simulink model "HEVModel"  (R2021a)
settings: Solver=ode4  StartTime=0  StopTime=tEnd  FixedStep=dt  RelTol=1e-3
values from neighbouring files (symbols this model uses):
  accessoryLoad = 600    [main.m]
  Af = 1.00    (= 1)    [main.m]
  batteryCapacity = 50    [main.m]
  batteryResistance = 0.0461    [main.m]
  C = 400    [main.m]
  Cd = 0.576    [main.m]
  Crr = 0.01    [main.m]
  cycleNum = 2    [main.m]
  EffTableEff = [.75 .85 .89 .95 .96 .97 .98 .99 .99]    [main.m]
  EffTableSpeed = [0 5 10 15 25 35 45 55 65]    [main.m]
  etaGenGR = 0.93    [main.m]
  g = 9.81    [main.m]
  genMotorData = load(GENERATOR_MOTOR_DATA_NAME)    [main.m]
  GRd = 9.843    [main.m]
  GRgen = 1.4    [main.m]
  initialGasVolume = 5    [main.m]
  k_gal2kWh = 32.3    [main.m]
  k_hr2s = 3600    [main.m]
  k_J2gal = 1/3600000/32.3    (= 8.59993120055e-09)    [main.m]
  k_kW2W = 1000    [main.m]
  k_kWh2J = 3.6*10^6    (= 3600000)    [main.m]
  k_m2mi = 0.000621371    [main.m]
  k_m32gal = 264.172    [main.m]
  k_rpm2rps = 2*pi()/60    [main.m]
  k_rps2rpm = 60/(2*pi)    (= 9.54929658551)    [main.m]
  k_s2h = 1/3600    (= 0.000277777777778)    [main.m]
  k_W2kW = 1/1000    (= 0.001)    [main.m]
  kc = 0.513    [main.m]
  Kd = 0    [main.m]
  Ki = 0.1    [main.m]
  ki = 0.0773    [main.m]
  Kp = 200    [main.m]
  kw = 0.0000064    (= 6.4e-06)    [main.m]
  m = 1965    [main.m]
  motorMaxPower = 310000    [main.m]
  motorMaxSpeed = 18000    [main.m]
  motorMaxTorque = 600    [main.m]
  openCircuitVoltage = 420    [main.m]
  pBrakeMax = 4*TbrakeMax / (mu_k*pi()* cylinderBore^2 *meanPadRadius*numPads)    [main.m]
  r = 0.290    (= 0.29)    [main.m]
  rho = 1.20    (= 1.2)    [main.m]
  SOCi = 90    [main.m]
  theta = 0    [main.m]
  v0 = 0    [main.m]
  x0 = 0    [main.m]
libraries: autolibshared x6, fl_lib x5, nesl_utility x5, sdl_lib x1, autolibsharedmappedengines x1
(part 1 of 3)
settings Model: Creator=Chris  LastModifiedBy=jordan
settings SolverCC: AlgebraicLoopSolver=TrustRegion
settings DebuggingCC: SFMachineParentedDataDiag=warning

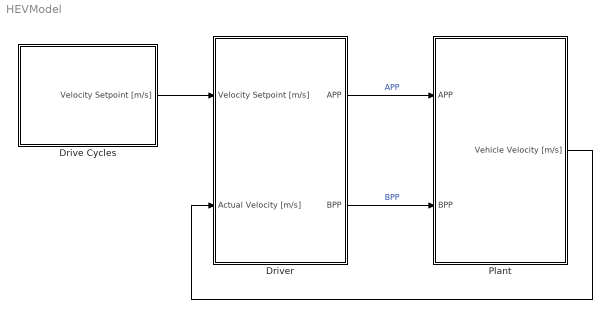
== system HEVModel ==
  Drive Cycles : Subsystem
  Driver : Subsystem
  Plant : Subsystem
  wires:
  Drive Cycles/1(Velocity Setpoint [m/s]) -> Driver/1(Velocity Setpoint [m/s])
  Driver/1(APP) -> Plant/1(APP)  "APP"
  Driver/2(BPP) -> Plant/2(BPP)  "BPP"
  Plant/1(Vehicle Velocity [m/s]) -> Driver/2(Actual Velocity [m/s])

== system HEVModel/Drive Cycles ==
  Constant : Constant  Value=cycleNum
  Drive Cycle Source1 : autolibshared/Drive Cycle Source  cycleVar=FTP75  wsVar=driveCycle  fileVar=cycleFTP75.mat  tfinal="2474  seconds"  cycleRepeat=off  outAccPort=off  outGearPort=off  gearList=No gear data  t_wot1=5  xdot_woto=0  xdot_wot1=30  t_wot2=20  xdot_wot2=0  t_wotend=30  srcUnit=m/s  outUnit=m/s  srcAccUnit=m/s/s  outAccUnit=m/s^2  dt=0  aMode=1  faultOption=off  velBnd=2  velBndUnit=mph  inUnit=m/s  timeBnd=1  failOption=off  stopSim=off  maxFaultCnt=10  maxFaultTime=2  maxTotFaultTime=15  traceOption=off  dtTrace=1  traceWindow=10  lastDCname=FTP75  lastOutUnit=mph  lastDT=0  lastTB=1  lastSB=2  forceCalcBound=off
      settings: SourceProductBaseCode=PW,DR,MT,UV,VE
  Drive Cycle Source2 : autolibshared/Drive Cycle Source  cycleVar=FTP75  wsVar=driveCycle  fileVar=cycleFTP75.mat  tfinal="2474  seconds"  cycleRepeat=off  outAccPort=off  outGearPort=off  gearList=No gear data  t_wot1=5  xdot_woto=0  xdot_wot1=30  t_wot2=20  xdot_wot2=0  t_wotend=30  srcUnit=m/s  outUnit=m/s  srcAccUnit=m/s/s  outAccUnit=m/s^2  dt=0  aMode=1  faultOption=off  velBnd=2  velBndUnit=mph  inUnit=m/s  timeBnd=1  failOption=off  stopSim=off  maxFaultCnt=10  maxFaultTime=2  maxTotFaultTime=15  traceOption=off  dtTrace=1  traceWindow=10  lastDCname=FTP75  lastOutUnit=mph  lastDT=0  lastTB=1  lastSB=2  forceCalcBound=off
      settings: SourceProductBaseCode=PW,DR,MT,UV,VE
  Drive Cycle Source3 : autolibshared/Drive Cycle Source  cycleVar=FTP75  wsVar=driveCycle  fileVar=cycleFTP75.mat  tfinal="2474  seconds, Cyclic"  cycleRepeat=on  outAccPort=off  outGearPort=off  gearList=No gear data  t_wot1=5  xdot_woto=0  xdot_wot1=30  t_wot2=20  xdot_wot2=0  t_wotend=30  srcUnit=m/s  outUnit=m/s  srcAccUnit=m/s/s  outAccUnit=m/s^2  dt=0  aMode=1  faultOption=off  velBnd=2  velBndUnit=mph  inUnit=m/s  timeBnd=1  failOption=off  stopSim=off  maxFaultCnt=10  maxFaultTime=2  maxTotFaultTime=15  traceOption=off  dtTrace=1  traceWindow=10  lastDCname=FTP75  lastOutUnit=mph  lastDT=0  lastTB=1  lastSB=2  forceCalcBound=off
      settings: SourceProductBaseCode=PW,DR,MT,UV,VE
  Drive Cycle Source4 : autolibshared/Drive Cycle Source  cycleVar=FTP75  wsVar=driveCycle  fileVar=cycleFTP75.mat  tfinal="2474  seconds, Cyclic"  cycleRepeat=on  outAccPort=off  outGearPort=off  gearList=No gear data  t_wot1=1  xdot_woto=0  xdot_wot1=30  t_wot2=tBrake  xdot_wot2=0  t_wotend=tWOTEnd  srcUnit=m/s  outUnit=m/s  srcAccUnit=m/s/s  outAccUnit=m/s^2  dt=0  aMode=1  faultOption=off  velBnd=2  velBndUnit=mph  inUnit=m/s  timeBnd=1  failOption=off  stopSim=off  maxFaultCnt=10  maxFaultTime=2  maxTotFaultTime=15  traceOption=off  dtTrace=1  traceWindow=10  lastDCname=FTP75  lastOutUnit=mph  lastDT=0  lastTB=1  lastSB=2  forceCalcBound=off
      settings: SourceProductBaseCode=PW,DR,MT,UV,VE
  Drive Cycle Source5 : autolibshared/Drive Cycle Source  cycleVar=FTP75  wsVar=driveCycle  fileVar=cycleFTP75.mat  tfinal="2474  seconds"  cycleRepeat=off  outAccPort=off  outGearPort=off  gearList=No gear data  t_wot1=5  xdot_woto=0  xdot_wot1=30  t_wot2=20  xdot_wot2=0  t_wotend=30  srcUnit=m/s  outUnit=m/s  srcAccUnit=m/s/s  outAccUnit=m/s^2  dt=0  aMode=1  faultOption=off  velBnd=2  velBndUnit=mph  inUnit=m/s  timeBnd=1  failOption=off  stopSim=off  maxFaultCnt=10  maxFaultTime=2  maxTotFaultTime=15  traceOption=off  dtTrace=1  traceWindow=10  lastDCname=FTP75  lastOutUnit=mph  lastDT=0  lastTB=1  lastSB=2  forceCalcBound=off
      settings: SourceProductBaseCode=PW,DR,MT,UV,VE
  Drive Cycle Source6 : autolibshared/Drive Cycle Source  cycleVar=Wide Open Throttle (WOT)  wsVar=driveCycle  fileVar=cycleFTP75.mat  tfinal="15  seconds, Cyclic"  cycleRepeat=on  outAccPort=off  outGearPort=off  gearList=No gear data  t_wot1=1  xdot_woto=0  xdot_wot1=vRef  t_wot2=tBrake2  xdot_wot2=-50  t_wotend=tEndWOT2  srcUnit=mph  outUnit=m/s  srcAccUnit=m/s/s  outAccUnit=m/s^2  dt=0  aMode=1  faultOption=off  velBnd=2  velBndUnit=mph  inUnit=m/s  timeBnd=1  failOption=off  stopSim=off  maxFaultCnt=10  maxFaultTime=2  maxTotFaultTime=15  traceOption=off  dtTrace=1  traceWindow=10  lastDCname=Custom Data Set  lastOutUnit=mph  lastDT=0  lastTB=1  lastSB=2  forceCalcBound=off
      settings: SourceProductBaseCode=PW,DR,MT,UV,VE
  Multiport Switch : MultiPortSwitch  Inputs=6
  Velocity Setpoint [m/s] : Outport
  wires:
  Drive Cycle Source6/1 -> Multiport Switch/7
  Drive Cycle Source5/1 -> Multiport Switch/6
  Drive Cycle Source4/1 -> Multiport Switch/4
  Drive Cycle Source1/1 -> Multiport Switch/5
  Drive Cycle Source2/1 -> Multiport Switch/2
  Constant/1 -> Multiport Switch/1
  Multiport Switch/1 -> Velocity Setpoint [m/s]/1  "Velocity Setpoint [m/s]"
  Drive Cycle Source3/1 -> Multiport Switch/3

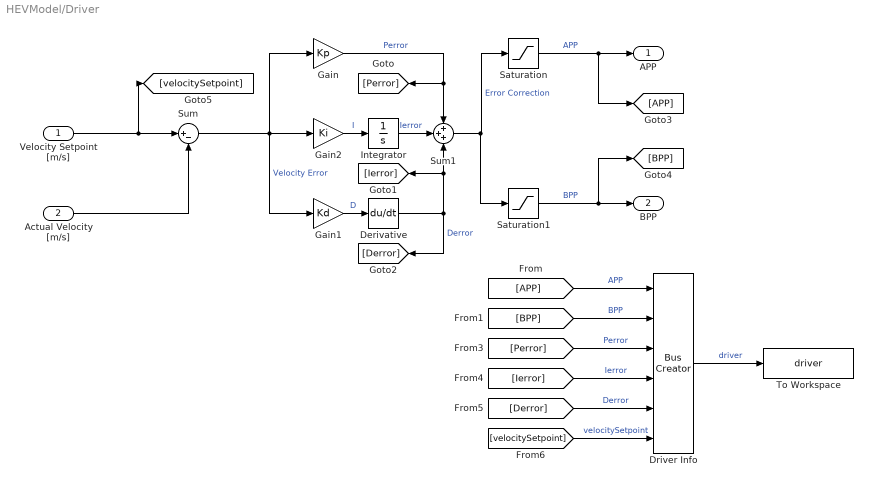
== system HEVModel/Driver ==
  Velocity Setpoint [m/s] : Inport
  Actual Velocity [m/s] : Inport  Port=2
  Derivative : Derivative
  Driver Info : BusCreator  Inputs=6
  Gain : Gain  Gain=Kp
  Gain1 : Gain  Gain=Kd
  Gain2 : Gain  Gain=Ki
  Integrator : Integrator
  Saturation : Saturate  UpperLimit=100  LowerLimit=0
  Saturation1 : Saturate  UpperLimit=0  LowerLimit=-100
  Sum : Sum  Inputs=|+-
  Sum1 : Sum  Inputs=+++
  To Workspace : ToWorkspace  VariableName=driver  SaveFormat=Timeseries  SampleTime=-1
  APP : Outport
  BPP : Outport  Port=2
  wires:
  Gain/1 -> [Perror], Sum1/1  "Perror"
  Integrator/1 -> Sum1/2  "Ierror"
  Derivative/1 -> [Derror], [Ierror], Sum1/3  "Derror"
  Sum1/1 -> Saturation1/1, Saturation/1  "Error Correction"
  Sum/1 -> Gain2/1, Gain1/1, Gain/1  "Velocity Error"
  Velocity Setpoint [m/s]/1 -> [velocitySetpoint], Sum/1
  Actual Velocity [m/s]/1 -> Sum/2
  Saturation1/1 -> [BPP], BPP/1  "BPP"
  Saturation/1 -> [APP], APP/1  "APP"
  Gain2/1 -> Integrator/1  "I"
  Gain1/1 -> Derivative/1  "D"
  Driver Info/1 -> To Workspace/1  "driver"
  [APP] -> Driver Info/1  "APP"
  [BPP] -> Driver Info/2  "BPP"
  [Perror] -> Driver Info/3  "Perror"
  [Ierror] -> Driver Info/4  "Ierror"
  [Derror] -> Driver Info/5  "Derror"
  [velocitySetpoint] -> Driver Info/6  "velocitySetpoint"

== system HEVModel/Plant ==
  APP : Inport
  BPP : Inport  Port=2
  Battery : Subsystem
  Brakes : Subsystem
  Driveline : Subsystem
  Fuel Tank Volume [gal] : Display
  Genset : Subsystem
  Motor : Subsystem
  State of Charge : Display
  Sum : Sum  Inputs=|-+
  "Thermostatic Hybrid Supervisory Controller " : Subsystem
  Vehicle Dynamics : Subsystem
  Vehicle Velocity [m/s] : Outport
  wires:
  APP/1 -> Motor/1(APP)
  Sum/1 -> Battery/1(Power to Motor [W])
  Motor/1(Motor Input Power [W]) -> Sum/2
  Motor/2(Motor Output Torque [Nm]) -> Driveline/1(Motor Torque [Nm])  "Motor Torque [Nm]"
  "Thermostatic Hybrid Supervisory Controller "/1(Engine Torque Command [Nm]) -> Genset/1(Engine Torque [Nm])
  Driveline/1(Wheel Torque [Nm]) -> Vehicle Dynamics/1(Wheel Torque [Nm])  "Wheel Torque [Nm]"
  Vehicle Dynamics/2(Wheel Angular Velocity [rad/s]) -> Brakes/2(Wheel Angular Velocity [rad/s])  "Wheel Angular Velocity [rad/s]"
  Brakes/1(Braking Torque [Nm]) -> Driveline/2(Braking Torque [Nm])  "Braking Torque [Nm]"
  Genset/2(Power Out [W]) -> Sum/1
  Vehicle Dynamics/1(Velocity [m/s]) -> Vehicle Velocity [m/s]/1  "Vehicle Velocity [m/s]"
  Genset/1(Fuel Tank Volume [gal]) -> "Thermostatic Hybrid Supervisory Controller "/1(Fuel Tank Volume [gal]), Fuel Tank Volume [gal]/1  "Fuel Tank Volume [gal]"
  BPP/1 -> Brakes/1(BPP)
  "Thermostatic Hybrid Supervisory Controller "/2(Motor Speed Command [rpm]) -> Genset/2(Motor Speed [rpm])
  Battery/1(SOC [%]) -> State of Charge/1, "Thermostatic Hybrid Supervisory Controller "/2(SOC [%])  "State of Charge"

== system HEVModel/Plant/Battery ==
  Power to Motor [W] : Inport
  Current Calculation : Subsystem
  Energy Calculations and Data Management : Subsystem
  SOC [%] : Outport
  wires:
  Power to Motor [W]/1 -> Current Calculation/1(Power to Motor [W])
  Energy Calculations and Data Management/1(SOC) -> SOC [%]/1

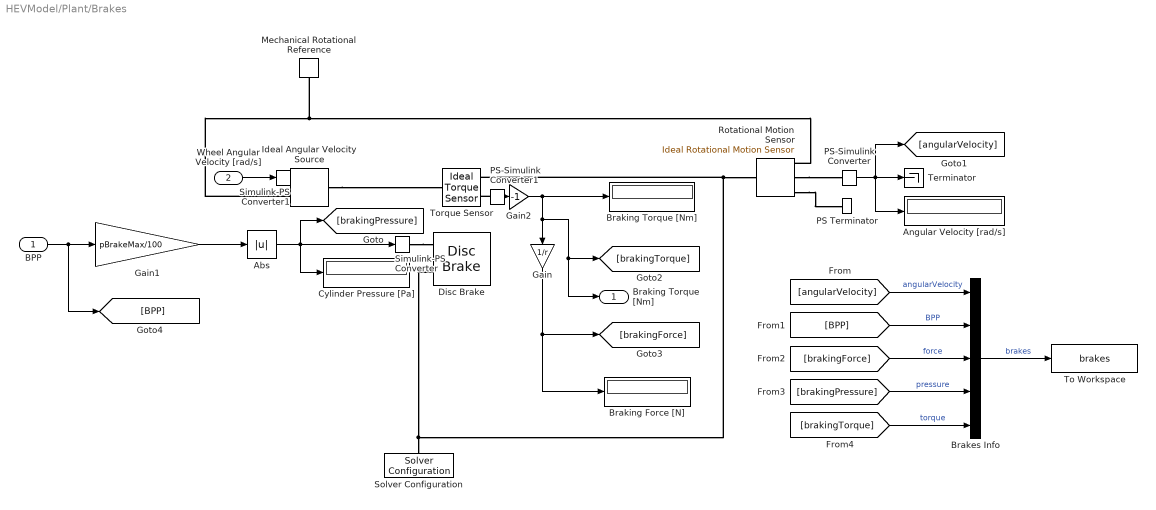
== system HEVModel/Plant/Brakes ==
  BPP : Inport
  Wheel Angular Velocity [rad/s] : Inport  Port=2
  Abs : Abs
  Angular Velocity [rad/s] : Display
  Brakes Info : BusCreator  Inputs=5
  Braking Force [N] : Display
  Braking Torque [Nm] : Display
  Cylinder Pressure [Pa] : Display
  Disc Brake : sdl_lib/Brakes & Detents/Rotational/Disc Brake  r_mean=meanPadRadius m  bore=cylinderBore m  n_pads=numPads  thermal_port=simscape.enum.thermaleffects.omit  mu_static=mu_s  mu_coulomb=mu_k  temperature_TLU=[280, 300, 320] K  mu_static_TLU=[.9, .8, .7]  mu_coulomb_TLU=[.8, .7, .6]  thermal_mass=50 kJ/K  brkwy_vel=omegaBreakAway rad/s  visc_coef=mu_v N*m/(rad/s)  enable_faults=simscape.enum.onoff.off  faulted_pressure=0 bar  external_fault=simscape.enum.onoff.off  temporal_fault=simscape.enum.onoff.off  fault_time=5 s  report_fault=simscape.enum.assert.action.none  temperature_specify=off  temperature_priority=High  temperature=300 K  temperature_nominal_specify=off  temperature_nominal_unit=K  temperature_nominal_value=1
      settings: SourceProductBaseCode=LD
  Gain : Gain  Gain=1/r
  Gain1 : Gain  Gain=pBrakeMax/100
  Gain2 : Gain  Gain=-1
  Ideal Angular Velocity Source : fl_lib/Mechanical/Mechanical Sources/Ideal Angular Velocity Source
  Mechanical Rotational Reference : fl_lib/Mechanical/Rotational Elements/Mechanical Rotational Reference
  PS Terminator : fl_lib/Physical Signals/Sinks/PS Terminator
  PS-Simulink Converter : nesl_utility/PS-Simulink Converter  PhysicalDomain=network_engine_domain  SubClassName=ps_output  LeftPortType=input  RightPortType=output  PseudoPeriodic=off  Frequencies=[]  Unit=inherit  AffineConversion=off
      settings: SourceProductBaseCode=PW,SS
  PS-Simulink Converter1 : nesl_utility/PS-Simulink Converter  PhysicalDomain=network_engine_domain  SubClassName=ps_output  LeftPortType=input  RightPortType=output  PseudoPeriodic=off  Frequencies=[]  Unit=inherit  AffineConversion=off
      settings: SourceProductBaseCode=PW,SS
  Rotational Motion Sensor : fl_lib/Mechanical/Mechanical Sensors/Ideal Rotational Motion Sensor  wrap_angle=simscape.enum.onoff.off  offset=0 rad
  Simulink-PS Converter : nesl_utility/Simulink-PS Converter  PhysicalDomain=network_engine_domain  SubClassName=ps_input  LeftPortType=input  RightPortType=output  PseudoPeriodic=off  Frequencies=[]  NoiseDistribution=none  NoiseParameters=[]  Unit=Pa  AffineConversion=off  FilteringAndDerivatives=provide  SimscapeFilterOrder=1  InputFilterTimeConstant=0.001  UdotUserProvided=0
      settings: SourceProductBaseCode=PW,SS
  Simulink-PS Converter1 : nesl_utility/Simulink-PS Converter  PhysicalDomain=network_engine_domain  SubClassName=ps_input  LeftPortType=input  RightPortType=output  PseudoPeriodic=off  Frequencies=[]  NoiseDistribution=none  NoiseParameters=[]  Unit=rad/s  AffineConversion=off  FilteringAndDerivatives=provide  SimscapeFilterOrder=1  InputFilterTimeConstant=0.001  UdotUserProvided=0
      settings: SourceProductBaseCode=PW,SS
  Solver Configuration : nesl_utility/Solver Configuration  PhysicalDomain=network_engine_domain  SubClassName=solver  LeftPortType=input  RightPortType=generic  Tones=[]  Harmonics=[]  SimulateNoise=off  Profile=off  UseLocalSampling=off  EnableSwitchedLinearOptims=on  FrequencyDomain=off  UseCCode=off  RelTol=0.001  AbsTol=1e-06  MinStep=1e-09  ToWorkspace=off  RevertToSquareIcSolve=off  NumHomotopyIterations=100  PhasorMode=off  PhasorModeNumHarmonics=1  DoDC=on  ResidualTolerance=1e-09  UseLocalSolver=on  LocalSolverChoice=NE_BACKWARD_EULER_ADVANCER  LocalSolverSampleTime=0.01  DoFixedCost=on  MaxNonlinIter=3  MaxModeIter=2  ComputeImpulses=off  ImpulseIterations=2  LinearAlgebra=auto  EquationFormulation=NE_TIME_EF  DelaysMemoryBudget=1024  AutomaticFiltering=on  FilteringTimeConstant=0.001  PartitionStorageMethod=AS_NEEDED  PartitionMemoryBudget=1024  PartitionMethod=ROBUST
      settings: SourceProductBaseCode=PW,SS
  Terminator : Terminator
  To Workspace : ToWorkspace  VariableName=brakes  SaveFormat=Timeseries  SampleTime=-1
  Torque Sensor : fl_lib/Mechanical/Mechanical Sensors/Ideal Torque Sensor
  Braking Torque [Nm] : Outport
  wires:
  Gain/1 -> Braking Force [N]/1, [brakingForce]
  Gain2/1 -> Braking Torque [Nm]/1, [brakingTorque], Braking Torque [Nm]/1, Gain/1
  PS-Simulink Converter/1 -> [angularVelocity], Angular Velocity [rad/s]/1, Terminator/1
  Abs/1 -> [brakingPressure], Cylinder Pressure [Pa]/1, Simulink-PS Converter/1
  Gain1/1 -> Abs/1
  BPP/1 -> [BPP], Gain1/1
  [angularVelocity] -> Brakes Info/1  "angularVelocity"
  [BPP] -> Brakes Info/2  "BPP"
  [brakingForce] -> Brakes Info/3  "force"
  [brakingPressure] -> Brakes Info/4  "pressure"
  [brakingTorque] -> Brakes Info/5  "torque"
  Brakes Info/1 -> To Workspace/1  "brakes"
  PS-Simulink Converter1/1 -> Gain2/1
  Wheel Angular Velocity [rad/s]/1 -> Simulink-PS Converter1/1
  connections:
  Simulink-PS Converter1/RConn1 -- Ideal Angular Velocity Source/RConn1
  Rotational Motion Sensor/RConn2 -- PS-Simulink Converter/LConn1
  Torque Sensor/RConn1 -- Rotational Motion Sensor/LConn1 -- Disc Brake/LConn2 -- Solver Configuration/RConn1
  Ideal Angular Velocity Source/RConn2 -- Rotational Motion Sensor/RConn1 -- Mechanical Rotational Reference/LConn1
  Ideal Angular Velocity Source/LConn1 -- Torque Sensor/LConn1
  Rotational Motion Sensor/RConn3 -- PS Terminator/LConn1
  Simulink-PS Converter/RConn1 -- Disc Brake/LConn1
  PS-Simulink Converter1/LConn1 -- Torque Sensor/RConn2

== system HEVModel/Plant/Driveline ==
  Motor Torque [Nm] : Inport
  Braking Torque [Nm] : Inport  Port=2
  Efficiency Look-up Table : Lookup_n-D  NumberOfTableDimensions=1  BreakpointsForDimension1=EffTableSpeed  Table=EffTableEff  InternalRulePriority=Speed  RndMeth=Simplest  InputSameDT=on
  Gain1 : Gain  Gain=GRd
  Product1 : Product
  Sum1 : Sum
  Wheel Torque [Nm] : Outport
  wires:
  Motor Torque [Nm]/1 -> Gain1/1
  Gain1/1 -> Product1/2  "Positive Torque [N-m]"
  Braking Torque [Nm]/1 -> Sum1/2  "Braking Torque [N-m]"
  Sum1/1 -> Wheel Torque [Nm]/1
  [velocityActual] -> Efficiency Look-up Table/1  "Velocity Actual [m/s]"
  Efficiency Look-up Table/1 -> Product1/1  "Driveline Efficiency"
  Product1/1 -> Sum1/1

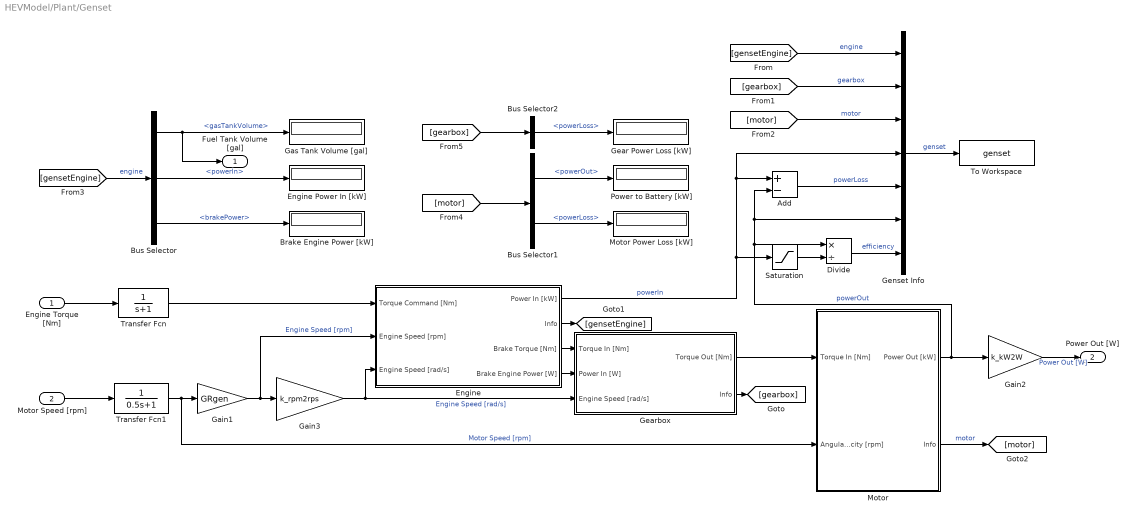
== system HEVModel/Plant/Genset ==
  Engine Torque [Nm] : Inport
  Motor Speed [rpm] : Inport  Port=2
  Add : Sum  Inputs=+-
  Brake Engine Power [kW] : Display
  Bus Selector : BusSelector  OutputSignals=gasTankVolume,powerIn,brakePower
  Bus Selector1 : BusSelector  OutputSignals=powerOut,powerLoss
  Bus Selector2 : BusSelector  OutputSignals=powerLoss
  Divide : Product  Inputs=*/
  Engine : Subsystem
  Engine Power In [kW] : Display
  Gain1 : Gain  Gain=GRgen
  Gain2 : Gain  Gain=k_kW2W
  Gain3 : Gain  Gain=k_rpm2rps
  Gas Tank Volume [gal] : Display
  Gear Power Loss [kW] : Display
  Gearbox : Subsystem
  Genset Info : BusCreator  Inputs=7
  Motor : Subsystem
  Motor Power Loss [kW] : Display
  Power to Battery [kW] : Display
  Saturation : Saturate  UpperLimit=inf  LowerLimit=eps
  To Workspace : ToWorkspace  VariableName=genset  SaveFormat=Timeseries  SampleTime=-1
  Transfer Fcn : TransferFcn  Denominator=[1 1]
  Transfer Fcn1 : TransferFcn  Denominator=[0.5 1]
  Fuel Tank Volume [gal] : Outport
  Power Out [W] : Outport  Port=2
  wires:
  Bus Selector/1 -> Fuel Tank Volume [gal]/1, Gas Tank Volume [gal]/1  "<gasTankVolume>"
  Motor Speed [rpm]/1 -> Transfer Fcn1/1
  Motor/2(Info) -> [motor]  "motor"
  [motor] -> Bus Selector1/1
  Bus Selector1/2 -> Motor Power Loss [kW]/1  "<powerLoss>"
  [gensetEngine] -> Bus Selector/1  "engine"
  Bus Selector2/1 -> Gear Power Loss [kW]/1  "<powerLoss>"
  Engine Torque [Nm]/1 -> Transfer Fcn/1
  Bus Selector/3 -> Brake Engine Power [kW]/1  "<brakePower>"
  Bus Selector1/1 -> Power to Battery [kW]/1  "<powerOut>"
  Engine/1(Power In [kW]) -> Saturation/1, Genset Info/4, Add/1  "powerIn"
  [gearbox] -> Bus Selector2/1
  Bus Selector/2 -> Engine Power In [kW]/1  "<powerIn>"
  Divide/1 -> Genset Info/7  "efficiency"
  Gain1/1 -> Engine/2(Engine Speed [rpm]), Gain3/1  "Engine Speed [rpm]"
  Transfer Fcn1/1 -> Motor/2(Angular Velocity [rpm]), Gain1/1  "Motor Speed [rpm]"
  Add/1 -> Genset Info/5  "powerLoss"
  Engine/3(Brake Torque [Nm]) -> Gearbox/1(Torque In [Nm])
  Gain3/1 -> Engine/3(Engine Speed [rad/s]), Gearbox/3(Engine Speed [rad/s])  "Engine Speed [rad/s]"
  Gearbox/1(Torque Out [Nm]) -> Motor/1(Torque In [Nm])
  [motor] -> Genset Info/3  "motor"
  [gearbox] -> Genset Info/2  "gearbox"
  Motor/1(Power Out [kW]) -> Gain2/1, Genset Info/6, Add/2, Divide/1  "powerOut"
  Gearbox/2(Info) -> [gearbox]
  [gensetEngine] -> Genset Info/1  "engine"
  Engine/2(Info) -> [gensetEngine]
  Genset Info/1 -> To Workspace/1  "genset"
  Engine/4(Brake Engine Power [W]) -> Gearbox/2(Power In [W])
  Transfer Fcn/1 -> Engine/1(Torque Command [Nm])
  Gain2/1 -> Power Out [W]/1  "Power Out [W]"
  Saturation/1 -> Divide/2

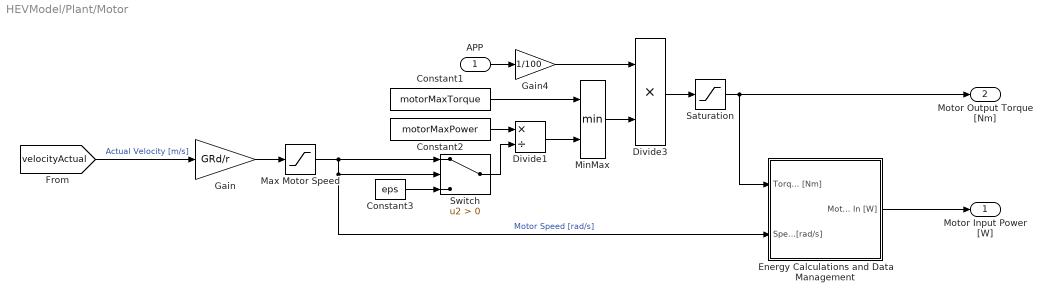
== system HEVModel/Plant/Motor ==
  APP : Inport
  Constant1 : Constant  Value=motorMaxTorque
  Constant2 : Constant  Value=motorMaxPower
  Constant3 : Constant  Value=eps
  Divide1 : Product  Inputs=*/
  Divide3 : Product  Inputs=**
  Energy Calculations and Data Management : Subsystem
  Gain : Gain  Gain=GRd/r
  Gain4 : Gain  Gain=1/100
  Max Motor Speed : Saturate  UpperLimit=motorMaxSpeed/k_rps2rpm  LowerLimit=0
  MinMax : MinMax  Inputs=2
  Saturation : Saturate  UpperLimit=motorMaxTorque  LowerLimit=0
  Switch : Switch  Criteria=u2 > Threshold
  Motor Input Power [W] : Outport
  Motor Output Torque [Nm] : Outport  Port=2
  wires:
  Gain/1 -> Max Motor Speed/1
  [velocityActual] -> Gain/1  "Actual Velocity [m/s]"
  APP/1 -> Gain4/1
  Constant1/1 -> MinMax/1
  Constant3/1 -> Switch/3
  Divide1/1 -> MinMax/2
  Divide3/1 -> Saturation/1
  Saturation/1 -> Motor Output Torque [Nm]/1, Energy Calculations and Data Management/1(Torque [Nm])
  Max Motor Speed/1 -> Energy Calculations and Data Management/2(Speed [rad/s]), Switch/2, Switch/1  "Motor Speed [rad/s]"
  Switch/1 -> Divide1/2
  Constant2/1 -> Divide1/1
  Gain4/1 -> Divide3/1
  MinMax/1 -> Divide3/2
  Energy Calculations and Data Management/1(Motor Power In [W]) -> Motor Input Power [W]/1

== system HEVModel/Plant/Thermostatic Hybrid Supervisory Controller  ==
  Fuel Tank Volume [gal] : Inport
  SOC [%] : Inport  Port=2
  Chart : Stateflow chart  TreatAsAtomicUnit=on
  Engine Torque Command [Nm] : Outport
  Motor Speed Command [rpm] : Outport  Port=2
  wires:
  Chart/1(EngineTorque) -> Engine Torque Command [Nm]/1
  Chart/2(MotorSpeed) -> Motor Speed Command [rpm]/1
  SOC [%]/1 -> Chart/1(SOC)
  Fuel Tank Volume [gal]/1 -> Chart/2(FuelTankVolume)

== system HEVModel/Plant/Vehicle Dynamics ==
  Wheel Torque [Nm] : Inport
  Data Management : Subsystem
  Dynamics Calculations : Subsystem
  Energy Calculations : Subsystem
  Velocity [m/s] : Outport
  Wheel Angular Velocity [rad/s] : Outport  Port=2
  wires:
  Wheel Torque [Nm]/1 -> Dynamics Calculations/1(Wheel Torque [Nm])  "Wheel Torque [Nm]"
  Dynamics Calculations/1(Tractive Force [N]) -> Energy Calculations/1(Tractive Force [N])
  Dynamics Calculations/2(Velocity [m/s]) -> Energy Calculations/2(Velocity [m/s]), Velocity [m/s]/1
  Dynamics Calculations/3(Rolling Resistance [N]) -> Energy Calculations/3(Rolling Resistance [N])
  Dynamics Calculations/4(Grade Force [N]) -> Energy Calculations/4(Grade Force [N])
  Dynamics Calculations/5(Drag Force [N]) -> Energy Calculations/5(Drag Force [N])
  Dynamics Calculations/6(Angular Velocity [rad/s]) -> Wheel Angular Velocity [rad/s]/1, Energy Calculations/6(Angular Velocity [rad/s])

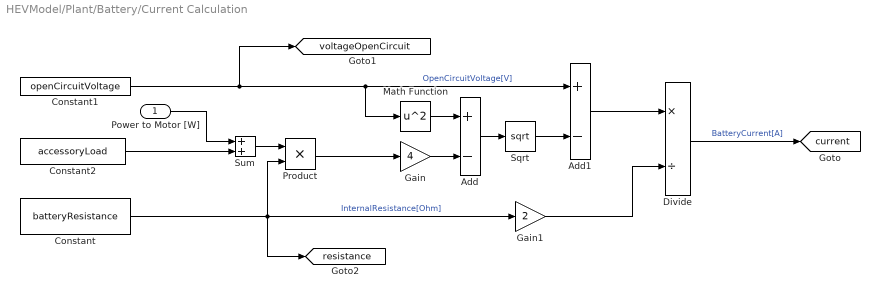
== system HEVModel/Plant/Battery/Current Calculation ==
  Power to Motor [W] : Inport
  Add : Sum  Inputs=+-
  Add1 : Sum  Inputs=+-
  Constant : Constant  Value=batteryResistance
  Constant1 : Constant  Value=openCircuitVoltage  SampleTime=-1
  Constant2 : Constant  Value=accessoryLoad
  Divide : Product  Inputs=*/
  Gain : Gain  Gain=4
  Gain1 : Gain  Gain=2
  Math Function : Math  Operator=square  SignedPower=on  SaturateOnIntegerOverflow=on
  Product : Product  RndMeth=Zero
  Sqrt : Sqrt  SaturateOnIntegerOverflow=on
  Sum : Sum
  tag scope: current=global, resistance=global, voltageOpenCircuit=global
  wires:
  Math Function/1 -> Add/1
  Gain/1 -> Add/2
  Add/1 -> Sqrt/1
  Constant/1 -> Product/2, Gain1/1, [resistance]  "InternalResistance[Ohm]"
  Sqrt/1 -> Add1/2
  Divide/1 -> [current]  "BatteryCurrent[A]"
  Power to Motor [W]/1 -> Sum/1
  Product/1 -> Gain/1
  Add1/1 -> Divide/1
  Gain1/1 -> Divide/2
  Constant1/1 -> Math Function/1, Add1/1, [voltageOpenCircuit]  "OpenCircuitVoltage[V]"
  Constant2/1 -> Sum/2
  Sum/1 -> Product/1

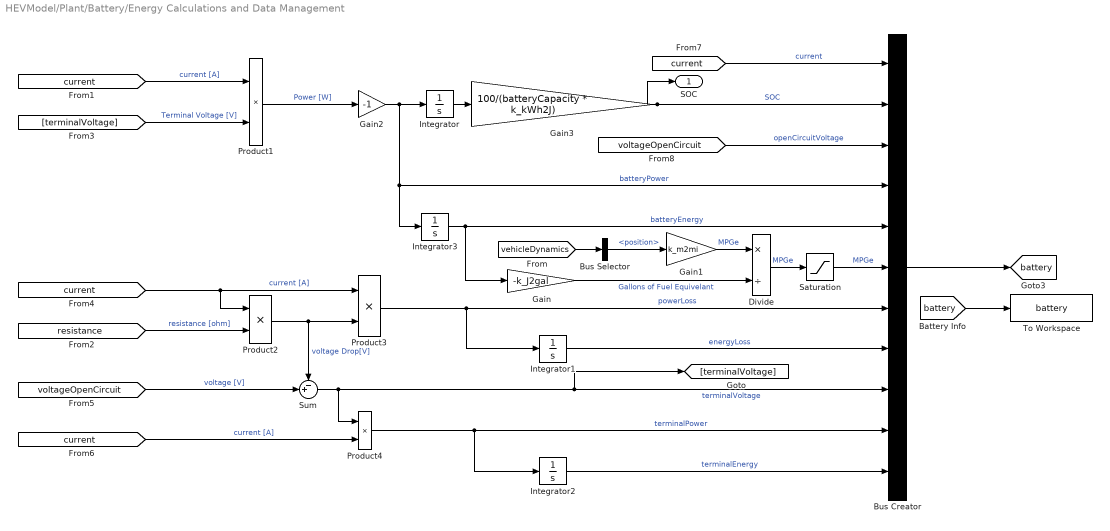
== system HEVModel/Plant/Battery/Energy Calculations and Data Management ==
  Bus Creator : BusCreator  Inputs=11
  Bus Selector : BusSelector  OutputSignals=position
  Divide : Product  Inputs=*/
  Gain : Gain  Gain=-k_J2gal
  Gain1 : Gain  Gain=k_m2mi
  Gain2 : Gain  Gain=-1
  Gain3 : Gain  Gain=100/(batteryCapacity * k_kWh2J)
  Integrator : Integrator  InitialCondition=(SOCi / 100) * batteryCapacity *k_kWh2J
  Integrator1 : Integrator
  Integrator2 : Integrator
  Integrator3 : Integrator
  Product1 : Product
  Product2 : Product
  Product3 : Product
  Product4 : Product  Inputs=**
  Saturation : Saturate  UpperLimit=300  LowerLimit=0
  Sum : Sum  Inputs=-+|
  To Workspace : ToWorkspace  VariableName=battery  SaveFormat=Timeseries  SampleTime=-1
  SOC : Outport
  tag scope: battery=global
  wires:
  Integrator/1 -> Gain3/1
  [current] -> Product1/1  "current [A]"
  Gain3/1 -> SOC/1, Bus Creator/2  "SOC"
  Integrator1/1 -> Bus Creator/8  "energyLoss"
  [current] -> Product3/1, Product2/1  "current [A]"
  Gain2/1 -> Bus Creator/4, Integrator3/1, Integrator/1  "batteryPower"
  Product1/1 -> Gain2/1  "Power [W]"
  Product4/1 -> Integrator2/1, Bus Creator/10  "terminalPower"
  [resistance] -> Product2/2  "resistance [ohm]"
  Product2/1 -> Product3/2, Sum/1  "voltage Drop[V]"
  Bus Creator/1 -> [battery]
  Product3/1 -> Bus Creator/7, Integrator1/1  "powerLoss"
  [voltageOpenCircuit] -> Sum/2  "voltage [V]"
  Sum/1 -> [terminalVoltage], Bus Creator/9, Product4/1  "terminalVoltage"
  [current] -> Bus Creator/1  "current"
  [current] -> Product4/2  "current [A]"
  Integrator2/1 -> Bus Creator/11  "terminalEnergy"
  [voltageOpenCircuit] -> Bus Creator/3  "openCircuitVoltage"
  Integrator3/1 -> Bus Creator/5, Gain/1  "batteryEnergy"
  [terminalVoltage] -> Product1/2  "Terminal Voltage [V]"
  Saturation/1 -> Bus Creator/6  "MPGe"
  [vehicleDynamics] -> Bus Selector/1
  Bus Selector/1 -> Gain1/1  "<position>"
  Gain1/1 -> Divide/1  "MPGe"
  Gain/1 -> Divide/2  "Gallons of Fuel Equivelant"
  [battery] -> To Workspace/1
  Divide/1 -> Saturation/1  "MPGe"
